simulink model "Control_deadbeat_sim"  (R2021a)
settings: Solver=VariableStepAuto  StartTime=0.0  StopTime=runTime  RelTol=1e-5  AbsTol=1e-5
values from neighbouring files (symbols this model uses):
  Cd = K*(1+1/(Ti*sd)+(Td*sd)/(1+Td*sd/N))    [ControlP.m]    (also in dead_2015.m = minreal(Fd/Pd/(1-Fd)); p4_3_diseño_directo.m = minreal(F/(Pd-F*Pd)))
  P = Km/(Tm*s+1)/(Tf*s+1)    [ControlP.m]    (also in ControlPID_RF.m; dead_2015.m; p4_3_diseño_directo.m = 20*(1-s)/(1+2*s)/(1+10*s))
  Pd = c2d(P,ts)    [ControlP.m]    (also in ControlPID_RF.m = -P; dead_2015.m = c2d(P, Ts, 'zoh'); p4_3_diseño_directo.m = c2d(P, Ts, 'zoh'))
  ts = 0.5    [ControlP.m]    (also in ControlPID_RF.m = 0.005; dead_2015.m = 0.055)
  Ts = ts    (= 0.5)    [ControlP.m]    (also in dead_2015.m = 0.055; p4_3_diseño_directo.m = 4.5)
settings Model: Creator=Fran  LastModifiedBy=Francisco

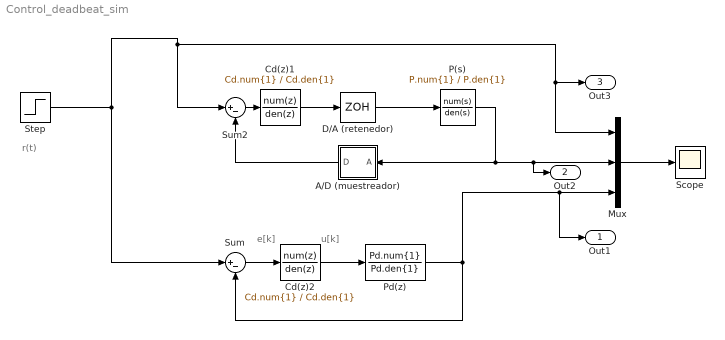
== system Control_deadbeat_sim ==
  note: r(t)
  note: u[k]
  note: e[k]
  A/D (muestreador) : Subsystem
  Cd(z)1 : DiscreteTransferFcn  Numerator=Cd.num{1}  Denominator=Cd.den{1}  SampleTime=ts
  Cd(z)2 : DiscreteTransferFcn  Numerator=Cd.num{1}  Denominator=Cd.den{1}  SampleTime=ts
  D/A (retenedor) : ZeroOrderHold  SampleTime=ts
  Mux : Mux  Inputs=3
  "P(s) " : TransferFcn  Numerator=P.num{1}  Denominator=P.den{1}
  Pd(z) : DiscreteTransferFcn  Numerator=Pd.num{1}  Denominator=Pd.den{1}  SampleTime=Ts
  Scope : Scope
  Step : Step  SampleTime=0
  Sum : Sum  Inputs=|+-
  Sum2 : Sum  Inputs=|+-
  Out1 : Outport  SignalName=Dig Exacto
  Out2 : Outport  Port=2  SignalName=Mixto
  Out3 : Outport  Port=3  SignalName=R
  wires:
  A/D (muestreador)/1(D) -> Sum2/2
  "P(s) "/1 -> Out2/1, Mux/2, A/D (muestreador)/1(A)
  Step/1 -> Out3/1, Mux/1, Sum2/1, Sum/1
  D/A (retenedor)/1 -> "P(s) "/1
  Sum2/1 -> Cd(z)1/1
  Cd(z)1/1 -> D/A (retenedor)/1
  Cd(z)2/1 -> Pd(z)/1
  Sum/1 -> Cd(z)2/1
  Pd(z)/1 -> Out1/1, Mux/3, Sum/2
  Mux/1 -> Scope/1

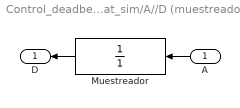
== system Control_deadbeat_sim/A//D (muestreador) ==
  A : Inport
  Muestreador : DiscreteTransferFcn  Numerator=1  Denominator=1  SampleTime=ts
  D : Outport
  wires:
  A/1 -> Muestreador/1
  Muestreador/1 -> D/1
